simulink model "BCM_C1A_EcuMonitor_4"  (Simulink 9.2)
settings: Solver=FixedStepDiscrete  StartTime=0.0  StopTime=5  FixedStep=0.01  RelTol=1e-3
undefined symbols (not defined in the file or in its folder): PRSK_DURATION_UNAVAILABLE_VALUE_CST, SECOND_TO_HUNDRED_MS_CST, TEN_CST, TYP_BCM_PRESOAK_REQUEST, TYP_HEVC_PRESOAK_ACTI_STATUS, TYP_LIN_LOW_LAYER, TYP_LOW_LAYER, TYP_RES_STATUS, TYP_UNDERHOOD_STATE, TYP_WAKE_UP_TYPE, ZERO_CST
libraries: Renault_Library x36, library_BCM x1
(part 1 of 2)
settings Model: Creator=p061584  LastModifiedBy=40005501
settings ConfigSet: Description=Test1
settings DataIOCC: SaveFormat=StructureWithTime  SignalLoggingSaveFormat=Dataset
settings DebuggingCC: SolverPrmCheckMsg=warning  InheritedTsInSrcMsg=none  ParameterPrecisionLossMsg=none
settings HardwareCC: ProdIntDivRoundTo=Zero  ProdEndianess=LittleEndian  ProdHWDeviceType=Generic->32-bit x86 compatible
settings SFSimCC: SimUseLocalCustomCode=on
settings RTWCC: RTWUseLocalCustomCode=on
settings GRTTargetCC: GeneratePreprocessorConditionals=Use local settings
settings ConfigComp: CovMetricSettings=dwe  CovHtmlReporting=off  CovSaveCumulativeToWorkspaceVar=off  CovSaveSingleToWorkspaceVar=off  CovExternalEMLEnable=on  DVMaxTestCaseSteps=500  DVTestSuiteOptimization=CombinedObjectives (Nonlinear Extended)  DVDetectDeadLogic=on  DVDetectActiveLogic=on  DVDetectOutOfBounds=on

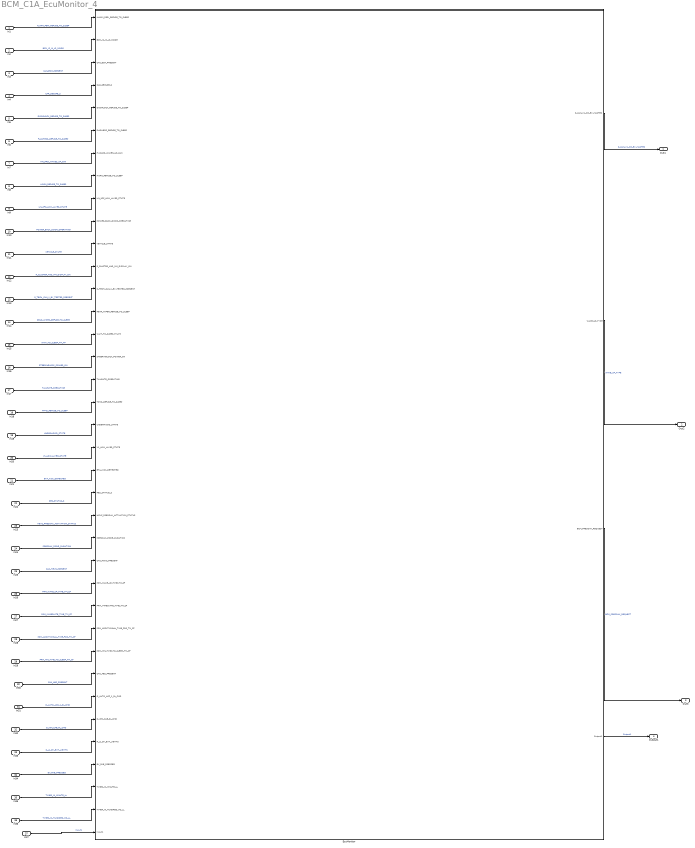
== system BCM_C1A_EcuMonitor_4 ==
  In1 : Inport
  In2 : Inport  Port=2
  In3 : Inport  Port=3
  In4 : Inport  Port=4
  In5 : Inport  Port=5
  In6 : Inport  Port=6
  In7 : Inport  Port=7
  In8 : Inport  Port=8
  In9 : Inport  Port=9
  In10 : Inport  Port=10
  In11 : Inport  Port=11
  In12 : Inport  Port=12
  In13 : Inport  Port=13
  In14 : Inport  Port=14
  In15 : Inport  Port=15
  In16 : Inport  Port=16
  In17 : Inport  Port=17
  In18 : Inport  Port=18
  In19 : Inport  Port=19
  In20 : Inport  Port=20
  In21 : Inport  Port=21
  In22 : Inport  Port=22
  In23 : Inport  Port=23
  In24 : Inport  Port=24
  In25 : Inport  Port=25
  In26 : Inport  Port=26
  In27 : Inport  Port=27
  In28 : Inport  Port=28
  In29 : Inport  Port=29
  In30 : Inport  Port=30
  In31 : Inport  Port=31
  In32 : Inport  Port=32
  In33 : Inport  Port=33
  In34 : Inport  Port=34
  In35 : Inport  Port=35
  In36 : Inport  Port=36
  In37 : Inport  Port=37  OutDataTypeStr=uint8
  EcuMonitor : Subsystem
  Out1 : Outport
  Out2 : Outport  Port=2
  Out3 : Outport  Port=3
  Output1 : Outport  Port=4  OutDataTypeStr=uint8
  wires:
  In30/1 -> EcuMonitor/30(CAN_ABS_PRESENT)  "CAN_ABS_PRESENT"
  In31/1 -> EcuMonitor/31(O_AUTO_ACC_1_RL_CMD)  "O_AUTO_ACC_1_RL_CMD"
  In22/1 -> EcuMonitor/22(RES_STATUS_S)  "RES_STATUS_S"
  In23/1 -> EcuMonitor/23(HEVC_PRESOAK_ACTIVATION_STATUS)  "HEVC_PRESOAK_ACTIVATION_STATUS"
  In24/1 -> EcuMonitor/24(PRESOAK_PROG_DURATION)  "PRESOAK_PROG_DURATION"
  In25/1 -> EcuMonitor/25(CAN_HEVC_PRESENT)  "CAN_HEVC_PRESENT"
  In26/1 -> EcuMonitor/26(PRM_WAKE_UP_TIME_TM_CF)  "PRM_WAKE_UP_TIME_TM_CF"
  In27/1 -> EcuMonitor/27(PRM_IMMEDIATE_TIME_TM_CF)  "PRM_IMMEDIATE_TIME_TM_CF"
  In28/1 -> EcuMonitor/28(PRM_ADDITIONNAL_TIME_FOR_TM_CF)  "PRM_ADDITIONNAL_TIME_FOR_TM_CF"
  In29/1 -> EcuMonitor/29(PRM_MIN_TIME_TO_SLEEP_TM_CF)  "PRM_MIN_TIME_TO_SLEEP_TM_CF"
  In32/1 -> EcuMonitor/32(O_IGN_CAB_RL_CMD)  "O_IGN_CAB_RL_CMD"
  In33/1 -> EcuMonitor/33(R_L1_BY_EXT_LIGHTS)  "R_L1_BY_EXT_LIGHTS"
  In34/1 -> EcuMonitor/34(EV_RKE_PRESSED)  "EV_RKE_PRESSED"
  In35/1 -> EcuMonitor/35(TIMER_IN_MINUTE_LL)  "TIMER_IN_MINUTE_LL"
  In36/1 -> EcuMonitor/36(TIMER_IN_HUNDRED_MS_LL)  "TIMER_IN_HUNDRED_MS_LL"
  In18/1 -> EcuMonitor/18(TPMS_REFUSE_TO_SLEEP)  "TPMS_REFUSE_TO_SLEEP"
  In19/1 -> EcuMonitor/19(UNDERHOOD_STATE)  "UNDERHOOD_STATE"
  In21/1 -> EcuMonitor/21(ETA_KICK_DETECTED)  "ETA_KICK_DETECTED"
  In1/1 -> EcuMonitor/1(ALARM_PERI_REFUSE_TO_SLEEP)  "ALARM_PERI_REFUSE_TO_SLEEP"
  In2/1 -> EcuMonitor/2(BCM_IS_IN_LP_MODE)  "BCM_IS_IN_LP_MODE"
  In3/1 -> EcuMonitor/3(CAN_ECM_PRESENT)  "CAN_ECM_PRESENT"
  In4/1 -> EcuMonitor/4(CAR_SECURE_S)  "CAR_SECURE_S"
  In5/1 -> EcuMonitor/5(DOORLOCK_REFUSE_TO_SLEEP)  "DOORLOCK_REFUSE_TO_SLEEP"
  In6/1 -> EcuMonitor/6(FLASHERS_REFUSE_TO_SLEEP)  "FLASHERS_REFUSE_TO_SLEEP"
  In7/1 -> EcuMonitor/7(HAZARD_WAKES_UP_CAN)  "HAZARD_WAKES_UP_CAN"
  In8/1 -> EcuMonitor/8(HORN_REFUSE_TO_SLEEP)  "HORN_REFUSE_TO_SLEEP"
  In9/1 -> EcuMonitor/9(LIN_NFC_LOW_LAYER_STATE)  "LIN_NFC_LOW_LAYER_STATE"
  In10/1 -> EcuMonitor/10(POWER_BACK_DOOR_OPERATING)  "POWER_BACK_DOOR_OPERATING"
  In11/1 -> EcuMonitor/11(VEHICLE_STATE)  "VEHICLE_STATE"
  In12/1 -> EcuMonitor/12(R_CLUSTER_AND_MM_DISPLAY_ON)  "R_CLUSTER_AND_MM_DISPLAY_ON"
  In13/1 -> EcuMonitor/13(R_TECH_CAN_V_BY_TESTER_PRESENT)  "R_TECH_CAN_V_BY_TESTER_PRESENT"
  In14/1 -> EcuMonitor/14(REAR_WIPER_REFUSE_TO_SLEEP)  "REAR_WIPER_REFUSE_TO_SLEEP"
  In15/1 -> EcuMonitor/15(WAIT_TO_SLEEP_TM_TP)  "WAIT_TO_SLEEP_TM_TP"
  In16/1 -> EcuMonitor/16(STEERINGLOCK_POWER_ON)  "STEERINGLOCK_POWER_ON"
  In17/1 -> EcuMonitor/17(TAILGATE_OPERATING)  "TAILGATE_OPERATING"
  EcuMonitor/1(R_CAN_V1_ON_BY_MASTER) -> Out1/1  "R_CAN_V1_ON_BY_MASTER"
  EcuMonitor/2(WAKE_UP_TYPE) -> Out2/1  "WAKE_UP_TYPE"
  EcuMonitor/3(BCM_PRESOAK_REQUEST) -> Out3/1  "BCM_PRESOAK_REQUEST"
  In20/1 -> EcuMonitor/20(V1_LOW_LAYER_STATE)  "V1_LOW_LAYER_STATE"
  In37/1 -> EcuMonitor/37(Input1)  "Input1"
  EcuMonitor/4(Output1) -> Output1/1  "Output1"

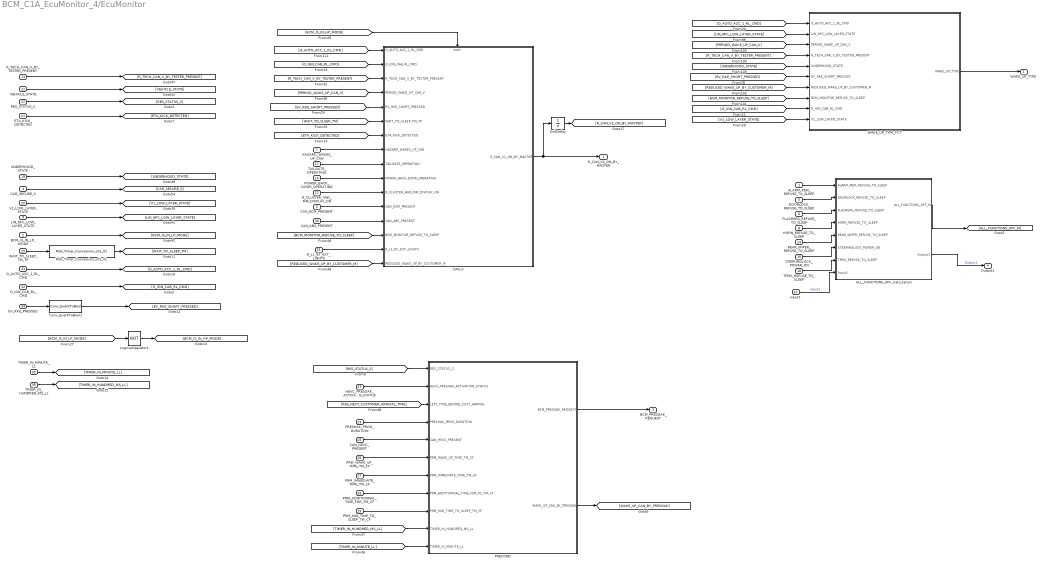
== system BCM_C1A_EcuMonitor_4/EcuMonitor ==
  ALARM_PERI_REFUSE_TO_SLEEP : Inport  OutDataTypeStr=boolean
  BCM_IS_IN_LP_MODE : Inport  Port=2  OutDataTypeStr=boolean
  CAN_ECM_PRESENT : Inport  Port=3  OutDataTypeStr=boolean
  CAR_SECURE_S : Inport  Port=4  OutDataTypeStr=boolean
  DOORLOCK_REFUSE_TO_SLEEP : Inport  Port=5  OutDataTypeStr=boolean
  FLASHERS_REFUSE_TO_SLEEP : Inport  Port=6  OutDataTypeStr=boolean
  HAZARD_WAKES_UP_CAN : Inport  Port=7  OutDataTypeStr=boolean
  HORN_REFUSE_TO_SLEEP : Inport  Port=8  OutDataTypeStr=boolean
  LIN_NFC_LOW_LAYER_STATE : Inport  Port=9  OutDataTypeStr=Enum: TYP_LIN_LOW_LAYER
  POWER_BACK_DOOR_OPERATING : Inport  Port=10  OutDataTypeStr=boolean
  VEHICLE_STATE : Inport  Port=11  OutDataTypeStr=Enum: TYP_VEHICLE_STATE
  R_CLUSTER_AND_MM_DISPLAY_ON : Inport  Port=12  OutDataTypeStr=boolean
  R_TECH_CAN_V_BY_TESTER_PRESENT : Inport  Port=13  OutDataTypeStr=boolean
  REAR_WIPER_REFUSE_TO_SLEEP : Inport  Port=14  OutDataTypeStr=boolean
  WAIT_TO_SLEEP_TM_TP : Inport  Port=15  OutDataTypeStr=uint16
  STEERINGLOCK_POWER_ON : Inport  Port=16  OutDataTypeStr=boolean
  TAILGATE_OPERATING : Inport  Port=17  OutDataTypeStr=boolean
  TPMS_REFUSE_TO_SLEEP : Inport  Port=18  OutDataTypeStr=boolean
  UNDERHOOD_STATE : Inport  Port=19  OutDataTypeStr=Enum: TYP_UNDERHOOD_STATE
  V1_LOW_LAYER_STATE : Inport  Port=20  OutDataTypeStr=Enum: TYP_LOW_LAYER
  ETA_KICK_DETECTED : Inport  Port=21  OutDataTypeStr=boolean
  RES_STATUS_S : Inport  Port=22  OutDataTypeStr=Enum: TYP_RES_STATUS
  HEVC_PRESOAK_ACTIVATION_STATUS : Inport  Port=23  OutDataTypeStr=Enum: TYP_HEVC_PRESOAK_ACTI_STATUS
      settings: AttributesFormatString=Type : %<OutDataTypeStr>
  PRESOAK_PROG_DURATION : Inport  Port=24  OutDataTypeStr=uint8
      settings: AttributesFormatString=Type : %<OutDataTypeStr>
  CAN_HEVC_PRESENT : Inport  Port=25  OutDataTypeStr=boolean
      settings: AttributesFormatString=Type : %<OutDataTypeStr>
  PRM_WAKE_UP_TIME_TM_CF : Inport  Port=26  OutDataTypeStr=uint16
      settings: AttributesFormatString=Type : %<OutDataTypeStr>
  PRM_IMMEDIATE_TIME_TM_CF : Inport  Port=27  OutDataTypeStr=uint16
      settings: AttributesFormatString=Type : %<OutDataTypeStr>
  PRM_ADDITIONNAL_TIME_FOR_TM_CF : Inport  Port=28  OutDataTypeStr=uint16
      settings: AttributesFormatString=Type : %<OutDataTypeStr>
  PRM_MIN_TIME_TO_SLEEP_TM_CF : Inport  Port=29  OutDataTypeStr=uint16
      settings: AttributesFormatString=Type : %<OutDataTypeStr>
  CAN_ABS_PRESENT : Inport  Port=30  OutDataTypeStr=boolean
  O_AUTO_ACC_1_RL_CMD : Inport  Port=31  OutDataTypeStr=boolean
  O_IGN_CAB_RL_CMD : Inport  Port=32  OutDataTypeStr=boolean
  R_L1_BY_EXT_LIGHTS : Inport  Port=33  OutDataTypeStr=boolean
  EV_RKE_PRESSED : Inport  Port=34  OutDataTypeStr=Enum: TYP_EVENT
  TIMER_IN_MINUTE_LL : Inport  Port=35  OutDataTypeStr=uint16
  TIMER_IN_HUNDRED_MS_LL : Inport  Port=36  OutDataTypeStr=uint16
      settings: AttributesFormatString=Type : %<OutDataTypeStr>
  Input1 : Inport  Port=37  OutDataTypeStr=uint8
  ALL_FUNCTIONS_OFF_Calculation : Subsystem
  CAN_V : Subsystem  Description=|
      | RQT_CAN_MANAGEMENT_BCM_420
      | RQT_CAN_MANAGEMENT_BCM_510
      | RQT_CAN_MANAGEMENT_BCM_520
      | RQT_CAN_MANAGEMENT_BCM_700
      | RQT_CAN_MANAGEMENT_BCM_716
      | RQT_EXTLIGHTS_BCM_40
      | RQT_BCM_CSV_4_0
  Conv_EventToBool1 : library_BCM/Modeling/Conv_EventToBool
  LogicalOperator1 : Logic  Operator=NOT  Inputs=7  OutDataTypeStr=boolean
  PRECOND : Subsystem  Description=<binary blob, 195 chars, not shown>
  RSA_Timer_Conversion_v01_01 : Renault_Library/Complex blocks/Timers & Counters/RSA_Timer_Conversion_v01_01  Tag=[LIB]  SAMPLE_TIME_CST=ECUMONITOR_SAMPLE_TIME_CST
      settings: AttributesFormatString=%<MaskType> : Ver : 01.01
  UnitDelay : UnitDelay  SampleTime=-1
      settings: AttributesFormatString=IC = %<X0>
  WAKE_UP_TYPE_FCT : Subsystem  Description=<binary blob, 216 chars, not shown>
  R_CAN_V1_ON_BY_MASTER : Outport  OutDataTypeStr=boolean
      settings: AttributesFormatString=Init :%<InitialOutput>
  WAKE_UP_TYPE : Outport  Port=2  OutDataTypeStr=Enum: TYP_WAKE_UP_TYPE
      settings: AttributesFormatString=Init :%<InitialOutput>
  BCM_PRESOAK_REQUEST : Outport  Port=3  OutDataTypeStr=Enum: TYP_BCM_PRESOAK_REQUEST
      settings: AttributesFormatString=Type : %<OutDataTypeStr>\nInit :%<InitialOutput>
  Output1 : Outport  Port=4  OutDataTypeStr=uint8
      settings: AttributesFormatString=Init :%<InitialOutput>
  wires:
  RES_STATUS_S/1 -> [RES_STATUS_S]
  CAN_ABS_PRESENT/1 -> CAN_V/13(CAN_ABS_PRESENT)
  CAN_ECM_PRESENT/1 -> CAN_V/12(CAN_ECM_PRESENT)
  ETA_KICK_DETECTED/1 -> [ETA_KICK_DETECTED]
  PRECOND/1(BCM_PRESOAK_REQUEST) -> BCM_PRESOAK_REQUEST/1
  PRM_MIN_TIME_TO_SLEEP_TM_CF/1 -> PRECOND/9(PRM_MIN_TIME_TO_SLEEP_TM_CF)
  HEVC_PRESOAK_ACTIVATION_STATUS/1 -> PRECOND/2(HEVC_PRESOAK_ACTIVATION_STATUS)
  [RES_NEXT_CUSTOMER_ARRIVAL_TIME] -> PRECOND/3(LEFT_TIME_BEFORE_CUST_ARRIVAL)
  PRESOAK_PROG_DURATION/1 -> PRECOND/4(PRESOAK_PROG_DURATION)
  CAN_HEVC_PRESENT/1 -> PRECOND/5(CAN_HEVC_PRESENT)
  [RES_STATUS_S] -> PRECOND/1(RES_STATUS_S)
  CAR_SECURE_S/1 -> [CAR_SECURE_S]
  [O_AUTO_ACC_1_RL_CMD] -> CAN_V/1(O_AUTO_ACC_1_RL_CMD)
  VEHICLE_STATE/1 -> [VEHICLE_STATE]
  WAKE_UP_TYPE_FCT/1(WAKE_UP_TYPE) -> WAKE_UP_TYPE/1
  [REDUCED_WAKE_UP_BY_CUSTOMER_M] -> WAKE_UP_TYPE_FCT/7(REDUCED_WAKE_UP_BY_CUSTOMER_M)
  [EV_RKE_SHORT_PRESSED] -> WAKE_UP_TYPE_FCT/6(EV_RKE_SHORT_PRESSED)
  [UNDERHOOD_STATE] -> WAKE_UP_TYPE_FCT/5(UNDERHOOD_STATE)
  [EV_RKE_SHORT_PRESSED] -> CAN_V/5(EV_RKE_SHORT_PRESSED)
  UNDERHOOD_STATE/1 -> [UNDERHOOD_STATE]
  [R_TECH_CAN_V_BY_TESTER_PRESENT] -> WAKE_UP_TYPE_FCT/4(R_TECH_CAN_V_BY_TESTER_PRESENT)
  [PERIOD_WAKE_UP_CAN_V] -> WAKE_UP_TYPE_FCT/3(PERIOD_WAKE_UP_CAN_V)
  [LIN_NFC_LOW_LAYER_STATE] -> WAKE_UP_TYPE_FCT/2(LIN_NFC_LOW_LAYER_STATE)
  [PERIOD_WAKE_UP_CAN_V] -> CAN_V/4(PERIOD_WAKE_UP_CAN_V)
  [R_TECH_CAN_V_BY_TESTER_PRESENT] -> CAN_V/3(R_TECH_CAN_V_BY_TESTER_PRESENT)
  R_TECH_CAN_V_BY_TESTER_PRESENT/1 -> [R_TECH_CAN_V_BY_TESTER_PRESENT]
  WAIT_TO_SLEEP_TM_TP/1 -> RSA_Timer_Conversion_v01_01/1
  R_CLUSTER_AND_MM_DISPLAY_ON/1 -> CAN_V/11(R_CLUSTER_AND_MM_DISPLAY_ON)
  BCM_IS_IN_LP_MODE/1 -> [BCM_IS_IN_LP_MODE]
  LIN_NFC_LOW_LAYER_STATE/1 -> [LIN_NFC_LOW_LAYER_STATE]
  V1_LOW_LAYER_STATE/1 -> [V1_LOW_LAYER_STATE]
  [ETA_KICK_DETECTED] -> CAN_V/7(ETA_KICK_DETECTED)
  CAN_V/1(R_CAN_V1_ON_BY_MASTER) -> UnitDelay/1, R_CAN_V1_ON_BY_MASTER/1
  HAZARD_WAKES_UP_CAN/1 -> CAN_V/8(HAZARD_WAKES_UP_CAN)
  TAILGATE_OPERATING/1 -> CAN_V/9(TAILGATE_OPERATING)
  POWER_BACK_DOOR_OPERATING/1 -> CAN_V/10(POWER_BACK_DOOR_OPERATING)
  PRECOND/2(WAKE_UP_CAN_BY_PRESOAK) -> [WAKE_UP_CAN_BY_PRESOAK]
  [WAIT_TO_SLEEP_TM] -> CAN_V/6(WAIT_TO_SLEEP_TM_TP)
  RSA_Timer_Conversion_v01_01/1 -> [WAIT_TO_SLEEP_TM]
  PRM_WAKE_UP_TIME_TM_CF/1 -> PRECOND/6(PRM_WAKE_UP_TIME_TM_CF)
  PRM_IMMEDIATE_TIME_TM_CF/1 -> PRECOND/7(PRM_IMMEDIATE_TIME_TM_CF)
  PRM_ADDITIONNAL_TIME_FOR_TM_CF/1 -> PRECOND/8(PRM_ADDITIONNAL_TIME_FOR_PC_TM_CF)
  O_AUTO_ACC_1_RL_CMD/1 -> [O_AUTO_ACC_1_RL_CMD]
  [O_AUTO_ACC_1_RL_CMD] -> WAKE_UP_TYPE_FCT/1(O_AUTO_ACC_1_RL_CMD)
  [O_IGN_CAB_RL_CMD] -> WAKE_UP_TYPE_FCT/9(O_IGN_CAB_RL_CMD)
  O_IGN_CAB_RL_CMD/1 -> [O_IGN_CAB_RL_CMD]
  [O_IGN_CAB_RL_CMD] -> CAN_V/2(O_IGN_CAB_RL_CMD)
  [BCM_MONITOR_REFUSE_TO_SLEEP] -> CAN_V/14(BCM_MONITOR_REFUSE_TO_SLEEP)
  R_L1_BY_EXT_LIGHTS/1 -> CAN_V/15(R_L1_BY_EXT_LIGHTS)
  EV_RKE_PRESSED/1 -> Conv_EventToBool1/1
  Conv_EventToBool1/1 -> [EV_RKE_SHORT_PRESSED]
  [BCM_IS_IN_LP_MODE] -> LogicalOperator1/1
  LogicalOperator1/1 -> [BCM_IS_IN_HP_MODE]
  [BCM_IS_IN_HP_MODE] -> CAN_V/Enable
  [REDUCED_WAKE_UP_BY_CUSTOMER_M] -> CAN_V/16(REDUCED_WAKE_UP_BY_CUSTOMER_M)
  [BCM_MONITOR_REFUSE_TO_SLEEP] -> WAKE_UP_TYPE_FCT/8(BCM_MONITOR_REFUSE_TO_SLEEP)
  ALARM_PERI_REFUSE_TO_SLEEP/1 -> ALL_FUNCTIONS_OFF_Calculation/1(ALARM_PERI_REFUSE_TO_SLEEP)
  DOORLOCK_REFUSE_TO_SLEEP/1 -> ALL_FUNCTIONS_OFF_Calculation/2(DOORLOCK_REFUSE_TO_SLEEP)
  FLASHERS_REFUSE_TO_SLEEP/1 -> ALL_FUNCTIONS_OFF_Calculation/3(FLASHERS_REFUSE_TO_SLEEP)
  HORN_REFUSE_TO_SLEEP/1 -> ALL_FUNCTIONS_OFF_Calculation/4(HORN_REFUSE_TO_SLEEP)
  REAR_WIPER_REFUSE_TO_SLEEP/1 -> ALL_FUNCTIONS_OFF_Calculation/5(REAR_WIPER_REFUSE_TO_SLEEP)
  STEERINGLOCK_POWER_ON/1 -> ALL_FUNCTIONS_OFF_Calculation/6(STEERINGLOCK_POWER_ON)
  TPMS_REFUSE_TO_SLEEP/1 -> ALL_FUNCTIONS_OFF_Calculation/7(TPMS_REFUSE_TO_SLEEP)
  ALL_FUNCTIONS_OFF_Calculation/1(ALL_FUNCTIONS_OFF_M) -> [ALL_FUNCTIONS_OFF_M]
  [V1_LOW_LAYER_STATE] -> WAKE_UP_TYPE_FCT/10(V1_LOW_LAYER_STATE)
  TIMER_IN_MINUTE_LL/1 -> [TIMER_IN_MINUTE_LL]
  TIMER_IN_HUNDRED_MS_LL/1 -> [TIMER_IN_HUNDRED_MS_LL]
  [TIMER_IN_HUNDRED_MS_LL] -> PRECOND/10(TIMER_IN_HUNDRED_MS_LL)
  [TIMER_IN_MINUTE_LL] -> PRECOND/11(TIMER_IN_MINUTE_LL)
  UnitDelay/1 -> [R_CAN_V1_ON_BY_MASTER]
  Input1/1 -> ALL_FUNCTIONS_OFF_Calculation/8(Input1)  "Input1"
  ALL_FUNCTIONS_OFF_Calculation/2(Output1) -> Output1/1  "Output1"

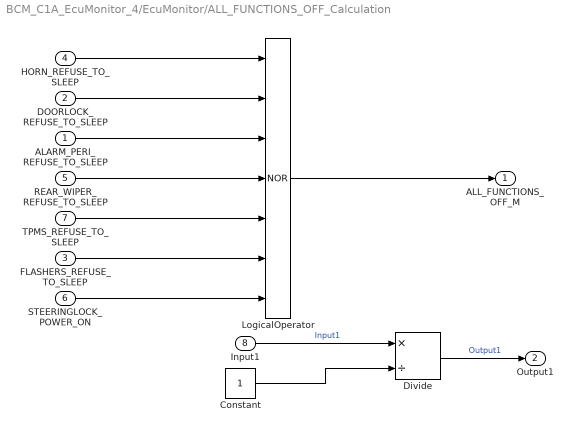
== system BCM_C1A_EcuMonitor_4/EcuMonitor/ALL_FUNCTIONS_OFF_Calculation ==
  ALARM_PERI_REFUSE_TO_SLEEP : Inport  OutDataTypeStr=boolean
  DOORLOCK_REFUSE_TO_SLEEP : Inport  Port=2  OutDataTypeStr=boolean
  FLASHERS_REFUSE_TO_SLEEP : Inport  Port=3  OutDataTypeStr=boolean
  HORN_REFUSE_TO_SLEEP : Inport  Port=4  OutDataTypeStr=boolean
  REAR_WIPER_REFUSE_TO_SLEEP : Inport  Port=5  OutDataTypeStr=boolean
  STEERINGLOCK_POWER_ON : Inport  Port=6  OutDataTypeStr=boolean
  TPMS_REFUSE_TO_SLEEP : Inport  Port=7  OutDataTypeStr=boolean
  Input1 : Inport  Port=8  OutDataTypeStr=uint8
  Constant : Constant
  Divide : Product  Inputs=*/  OutDataTypeStr=uint8
  LogicalOperator : Logic  Operator=NOR  Inputs=7  OutDataTypeStr=boolean
  ALL_FUNCTIONS_OFF_M : Outport
      settings: AttributesFormatString=Init :%<InitialOutput>
  Output1 : Outport  Port=2  OutDataTypeStr=uint8
      settings: AttributesFormatString=Init :%<InitialOutput>
  wires:
  LogicalOperator/1 -> ALL_FUNCTIONS_OFF_M/1
  STEERINGLOCK_POWER_ON/1 -> LogicalOperator/7
  FLASHERS_REFUSE_TO_SLEEP/1 -> LogicalOperator/6
  TPMS_REFUSE_TO_SLEEP/1 -> LogicalOperator/5
  REAR_WIPER_REFUSE_TO_SLEEP/1 -> LogicalOperator/4
  ALARM_PERI_REFUSE_TO_SLEEP/1 -> LogicalOperator/3
  DOORLOCK_REFUSE_TO_SLEEP/1 -> LogicalOperator/2
  HORN_REFUSE_TO_SLEEP/1 -> LogicalOperator/1
  Input1/1 -> Divide/1  "Input1"
  Constant/1 -> Divide/2
  Divide/1 -> Output1/1  "Output1"

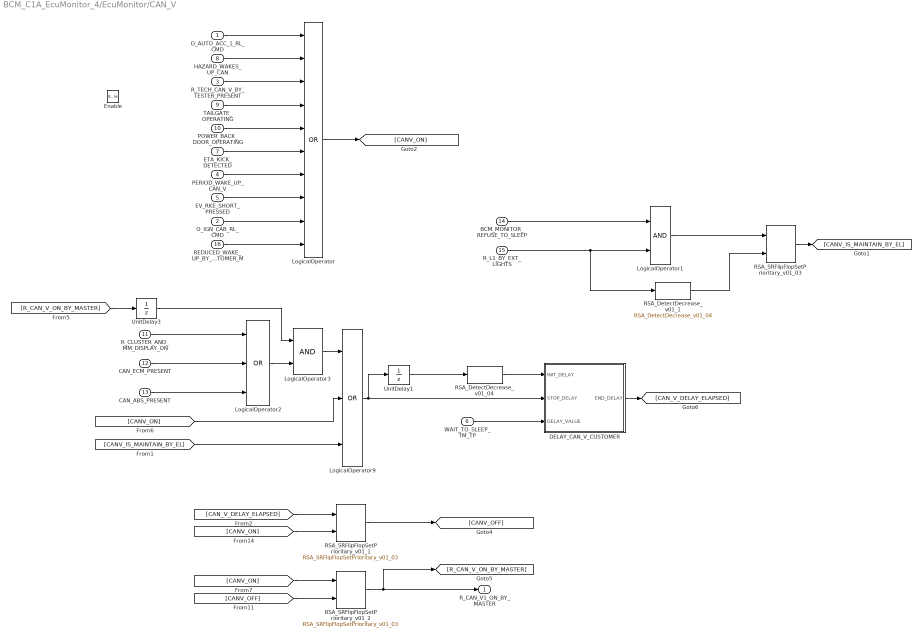
== system BCM_C1A_EcuMonitor_4/EcuMonitor/CAN_V ==
  O_AUTO_ACC_1_RL_CMD : Inport
      settings: AttributesFormatString=Type : %<OutDataTypeStr>
  O_IGN_CAB_RL_CMD : Inport  Port=2
      settings: AttributesFormatString=Type : %<OutDataTypeStr>
  R_TECH_CAN_V_BY_TESTER_PRESENT : Inport  Port=3
      settings: AttributesFormatString=Type : %<OutDataTypeStr>
  PERIOD_WAKE_UP_CAN_V : Inport  Port=4
      settings: AttributesFormatString=Type : %<OutDataTypeStr>
  EV_RKE_SHORT_PRESSED : Inport  Port=5
      settings: AttributesFormatString=Type : %<OutDataTypeStr>
  WAIT_TO_SLEEP_TM_TP : Inport  Port=6
      settings: AttributesFormatString=Type : %<OutDataTypeStr>
  ETA_KICK_DETECTED : Inport  Port=7
      settings: AttributesFormatString=Type : %<OutDataTypeStr>
  HAZARD_WAKES_UP_CAN : Inport  Port=8
      settings: AttributesFormatString=Type : %<OutDataTypeStr>
  TAILGATE_OPERATING : Inport  Port=9
      settings: AttributesFormatString=Type : %<OutDataTypeStr>
  POWER_BACK_DOOR_OPERATING : Inport  Port=10
      settings: AttributesFormatString=Type : %<OutDataTypeStr>
  R_CLUSTER_AND_MM_DISPLAY_ON : Inport  Port=11
      settings: AttributesFormatString=Type : %<OutDataTypeStr>
  CAN_ECM_PRESENT : Inport  Port=12
      settings: AttributesFormatString=Type : %<OutDataTypeStr>
  CAN_ABS_PRESENT : Inport  Port=13
      settings: AttributesFormatString=Type : %<OutDataTypeStr>
  BCM_MONITOR_REFUSE_TO_SLEEP : Inport  Port=14
      settings: AttributesFormatString=Type : %<OutDataTypeStr>
  R_L1_BY_EXT_LIGHTS : Inport  Port=15
      settings: AttributesFormatString=Type : %<OutDataTypeStr>
  REDUCED_WAKE_UP_BY_CUSTOMER_M : Inport  Port=16
      settings: AttributesFormatString=Type : %<OutDataTypeStr>
  Enable : EnablePort
      settings: AttributesFormatString=State : %<StatesWhenEnabling>
  DELAY_CAN_V_CUSTOMER : Subsystem
  LogicalOperator : Logic  Operator=OR  Inputs=10  OutDataTypeStr=boolean
  LogicalOperator1 : Logic  OutDataTypeStr=boolean
  LogicalOperator2 : Logic  Operator=OR  Inputs=3  OutDataTypeStr=boolean
  LogicalOperator3 : Logic  OutDataTypeStr=boolean
  LogicalOperator9 : Logic  Operator=OR  Inputs=3  OutDataTypeStr=boolean
  RSA_DetectDecrease_v01_04 : Renault_Library/Complex blocks/Logic & Bit Operations/RSA_DetectDecrease_v01_04  Tag=[LIB]  chkini=on  vinit=0
      settings: AttributesFormatString=%<MaskType> : Ver : 01.04\nCompare the Input with Initial Value = %<chkini>\nInitial Value : = %<vinit>
  RSA_DetectDecrease_v01_1 : Renault_Library/Complex blocks/Logic & Bit Operations/RSA_DetectDecrease_v01_04  Tag=[LIB]  chkini=on  vinit=0
      settings: AttributesFormatString=%<MaskType> : Ver : 01.04\nCompare the Input with Initial Value = %<chkini>\nInitial Value : = %<vinit>
  RSA_SRFlipFlopSetPrioritary_v01_03 : Renault_Library/Complex blocks/Flip-Flop/RSA_SRFlipFlopSetPrioritary_v01_03  Tag=[LIB]  init=false
      settings: AttributesFormatString=%<MaskType> : Ver : 01.03\n<init=%<init>>
  RSA_SRFlipFlopSetPrioritary_v01_1 : Renault_Library/Complex blocks/Flip-Flop/RSA_SRFlipFlopSetPrioritary_v01_03  Tag=[LIB]  init=false
      settings: AttributesFormatString=%<MaskType> : Ver : 01.03\n<init=%<init>>
  RSA_SRFlipFlopSetPrioritary_v01_2 : Renault_Library/Complex blocks/Flip-Flop/RSA_SRFlipFlopSetPrioritary_v01_03  Tag=[LIB]  init=false
      settings: AttributesFormatString=%<MaskType> : Ver : 01.03\n<init=%<init>>
  UnitDelay1 : UnitDelay  InitialCondition=false  SampleTime=-1
      settings: AttributesFormatString=IC = %<X0>
  UnitDelay3 : UnitDelay  InitialCondition=false  SampleTime=-1
      settings: AttributesFormatString=IC = %<X0>
  R_CAN_V1_ON_BY_MASTER : Outport
      settings: AttributesFormatString=Type : %<OutDataTypeStr>\nInit :%<InitialOutput>
  wires:
  O_AUTO_ACC_1_RL_CMD/1 -> LogicalOperator/1
  [CAN_V_DELAY_ELAPSED] -> RSA_SRFlipFlopSetPrioritary_v01_1/1
  LogicalOperator/1 -> [CANV_ON]
  RSA_SRFlipFlopSetPrioritary_v01_1/1 -> [CANV_OFF]
  [CANV_ON] -> RSA_SRFlipFlopSetPrioritary_v01_1/2
  [CANV_OFF] -> RSA_SRFlipFlopSetPrioritary_v01_2/2
  [CANV_ON] -> RSA_SRFlipFlopSetPrioritary_v01_2/1
  HAZARD_WAKES_UP_CAN/1 -> LogicalOperator/2
  R_TECH_CAN_V_BY_TESTER_PRESENT/1 -> LogicalOperator/3
  TAILGATE_OPERATING/1 -> LogicalOperator/4
  DELAY_CAN_V_CUSTOMER/1(END_DELAY) -> [CAN_V_DELAY_ELAPSED]
  WAIT_TO_SLEEP_TM_TP/1 -> DELAY_CAN_V_CUSTOMER/3(DELAY_VALUE)
  RSA_DetectDecrease_v01_04/1 -> DELAY_CAN_V_CUSTOMER/1(INIT_DELAY)
  [CANV_ON] -> LogicalOperator9/2
  [R_CAN_V_ON_BY_MASTER] -> UnitDelay3/1
  LogicalOperator9/1 -> UnitDelay1/1, DELAY_CAN_V_CUSTOMER/2(STOP_DELAY)
  UnitDelay1/1 -> RSA_DetectDecrease_v01_04/1
  LogicalOperator3/1 -> LogicalOperator9/1
  LogicalOperator2/1 -> LogicalOperator3/2
  CAN_ECM_PRESENT/1 -> LogicalOperator2/2
  CAN_ABS_PRESENT/1 -> LogicalOperator2/3
  R_CLUSTER_AND_MM_DISPLAY_ON/1 -> LogicalOperator2/1
  POWER_BACK_DOOR_OPERATING/1 -> LogicalOperator/5
  ETA_KICK_DETECTED/1 -> LogicalOperator/6
  PERIOD_WAKE_UP_CAN_V/1 -> LogicalOperator/7
  EV_RKE_SHORT_PRESSED/1 -> LogicalOperator/8
  RSA_SRFlipFlopSetPrioritary_v01_2/1 -> [R_CAN_V_ON_BY_MASTER], R_CAN_V1_ON_BY_MASTER/1
  UnitDelay3/1 -> LogicalOperator3/1
  O_IGN_CAB_RL_CMD/1 -> LogicalOperator/9
  R_L1_BY_EXT_LIGHTS/1 -> RSA_DetectDecrease_v01_1/1, LogicalOperator1/2
  BCM_MONITOR_REFUSE_TO_SLEEP/1 -> LogicalOperator1/1
  LogicalOperator1/1 -> RSA_SRFlipFlopSetPrioritary_v01_03/1
  RSA_SRFlipFlopSetPrioritary_v01_03/1 -> [CANV_IS_MAINTAIN_BY_EL]
  RSA_DetectDecrease_v01_1/1 -> RSA_SRFlipFlopSetPrioritary_v01_03/2
  [CANV_IS_MAINTAIN_BY_EL] -> LogicalOperator9/3
  REDUCED_WAKE_UP_BY_CUSTOMER_M/1 -> LogicalOperator/10

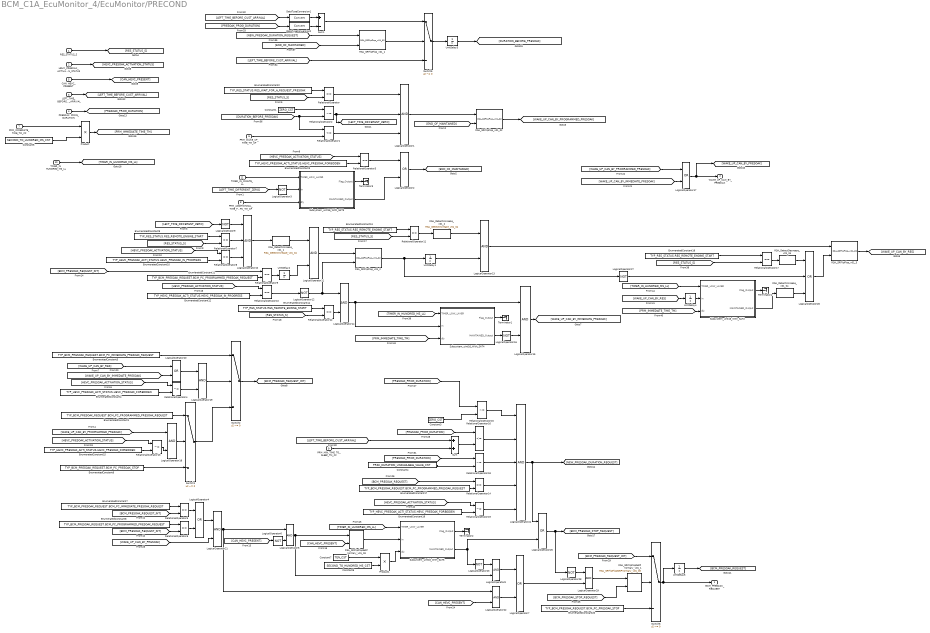
== system BCM_C1A_EcuMonitor_4/EcuMonitor/PRECOND ==
  RES_STATUS_S : Inport
      settings: AttributesFormatString=Type : %<OutDataTypeStr>
  HEVC_PRESOAK_ACTIVATION_STATUS : Inport  Port=2
      settings: AttributesFormatString=Type : %<OutDataTypeStr>
  LEFT_TIME_BEFORE_CUST_ARRIVAL : Inport  Port=3
      settings: AttributesFormatString=Type : %<OutDataTypeStr>
  PRESOAK_PROG_DURATION : Inport  Port=4
      settings: AttributesFormatString=Type : %<OutDataTypeStr>
  CAN_HEVC_PRESENT : Inport  Port=5
      settings: AttributesFormatString=Type : %<OutDataTypeStr>
  PRM_WAKE_UP_TIME_TM_CF : Inport  Port=6
      settings: AttributesFormatString=Type : %<OutDataTypeStr>
  PRM_IMMEDIATE_TIME_TM_CF : Inport  Port=7
      settings: AttributesFormatString=Type : %<OutDataTypeStr>
  PRM_ADDITIONNAL_TIME_FOR_PC_TM_CF : Inport  Port=8
      settings: AttributesFormatString=Type : %<OutDataTypeStr>
  PRM_MIN_TIME_TO_SLEEP_TM_CF : Inport  Port=9
      settings: AttributesFormatString=Type : %<OutDataTypeStr>
  TIMER_IN_HUNDRED_MS_LL : Inport  Port=10
      settings: AttributesFormatString=Type : %<OutDataTypeStr>
  TIMER_IN_MINUTE_LL : Inport  Port=11
      settings: AttributesFormatString=Type : %<OutDataTypeStr>
  Constant1 : Constant  Value=ZERO_CST  OutDataTypeStr=Inherit: Inherit via back propagation
  Constant3 : Constant  Value=ZERO_CST  OutDataTypeStr=uint8  SampleTime=-1
  Constant4 : Constant  Value=PRSK_DURATION_UNAVAILABLE_VALUE_CST  OutDataTypeStr=Inherit: Inherit via back propagation  SampleTime=-1
  Constant5 : Constant  Value=SECOND_TO_HUNDRED_MS_CST  OutDataTypeStr=uint16  SampleTime=-1
  Constant6 : Constant  Value=SECOND_TO_HUNDRED_MS_CST  OutDataTypeStr=uint16  SampleTime=-1
  Constant7 : Constant  Value=TEN_CST  OutDataTypeStr=uint16  SampleTime=-1
  DataTypeConversion1 : DataTypeConversion  RndMeth=Zero
      settings: AttributesFormatString=Saturation:%<SaturateOnIntegerOverflow>
  DataTypeConversion2 : DataTypeConversion  RndMeth=Zero
      settings: AttributesFormatString=Saturation:%<SaturateOnIntegerOverflow>
  EnumeratedConstant{1,8,11,17} (4 alike) : Constant  Value=TYP_BCM_PRESOAK_REQUEST.BCM_PC_PROGRAMMED_PRESOAK_REQUEST  OutDataTypeStr=Enum: TYP_BCM_PRESOAK_REQUEST  SampleTime=-1
  EnumeratedConstant10 : Constant  Value=TYP_HEVC_PRESOAK_ACTI_STATUS.HEVC_PRESOAK_IN_PROGRESS  OutDataTypeStr=Enum: TYP_HEVC_PRESOAK_ACTI_STATUS  SampleTime=-1
  EnumeratedConstant12 : Constant  Value=TYP_HEVC_PRESOAK_ACTI_STATUS.HEVC_PRESOAK_IN_PROGRESS  OutDataTypeStr=Enum: TYP_HEVC_PRESOAK_ACTI_STATUS  SampleTime=-1
  EnumeratedConstant{9,13..14,18} (4 alike) : Constant  Value=TYP_RES_STATUS.RES_REMOTE_ENGINE_START  OutDataTypeStr=Enum: TYP_RES_STATUS  SampleTime=-1
  EnumeratedConstant{3..4,15,19} (4 alike) : Constant  Value=TYP_HEVC_PRESOAK_ACTI_STATUS.HEVC_PRESOAK_FORBIDDEN  OutDataTypeStr=Enum: TYP_HEVC_PRESOAK_ACTI_STATUS  SampleTime=-1
  EnumeratedConstant2 : Constant  Value=TYP_RES_STATUS.RES_WAIT_FOR_A_REQUEST_PRESOAK  OutDataTypeStr=Enum: TYP_RES_STATUS  SampleTime=-1
  EnumeratedConstant20 : Constant  Value=TYP_BCM_PRESOAK_REQUEST.BCM_PC_PRESOAK_STOP  OutDataTypeStr=Enum: TYP_BCM_PRESOAK_REQUEST  SampleTime=-1
  EnumeratedConstant5 : Constant  Value=TYP_BCM_PRESOAK_REQUEST.BCM_PC_IMMEDIATE_PRESOAK_REQUEST  OutDataTypeStr=Enum: TYP_BCM_PRESOAK_REQUEST  SampleTime=-1
  EnumeratedConstant6 : Constant  Value=TYP_BCM_PRESOAK_REQUEST.BCM_PC_PRESOAK_STOP  OutDataTypeStr=Enum: TYP_BCM_PRESOAK_REQUEST  SampleTime=-1
  EnumeratedConstant7 : Constant  Value=TYP_BCM_PRESOAK_REQUEST.BCM_PC_IMMEDIATE_PRESOAK_REQUEST  OutDataTypeStr=Enum: TYP_BCM_PRESOAK_REQUEST  SampleTime=-1
  LogicalOperator1 : Logic  Inputs=3  OutDataTypeStr=boolean
  LogicalOperator10 : Logic  Inputs=3  OutDataTypeStr=boolean
  LogicalOperator{5,8,11,13..15,18..19,21..22,29} (11 alike) : Logic  OutDataTypeStr=boolean
  LogicalOperator{3,6,9,12,16,23,27..28} (8 alike) : Logic  Operator=NOT  OutDataTypeStr=boolean
  LogicalOperator{2,4,7,17,20,25} (6 alike) : Logic  Operator=OR  OutDataTypeStr=boolean
  LogicalOperator24 : Logic  Inputs=5  OutDataTypeStr=boolean
  LogicalOperator26 : Logic  Operator=OR  Inputs=3  OutDataTypeStr=boolean
  Product : Product  OutDataTypeStr=Inherit: Inherit via back propagation  RndMeth=Zero
  Product1 : Product  OutDataTypeStr=Inherit: Inherit via back propagation  RndMeth=Zero
  RSA_DetectDecrease_v01_04 : Renault_Library/Complex blocks/Logic & Bit Operations/RSA_DetectDecrease_v01_04  Tag=[LIB]  chkini=on  vinit=0
      settings: AttributesFormatString=%<MaskType> : Ver : 01.04\nCompare the Input with Initial Value = %<chkini>\nInitial Value : = %<vinit>
  RSA_DetectIncrease_v01_04 : Renault_Library/Complex blocks/Logic & Bit Operations/RSA_DetectIncrease_v01_04  Tag=[LIB]  chkini=on  vinit=0
      settings: AttributesFormatString=%<MaskType> : Ver : 01.04\nCompare the Input with Initial Value = %<chkini>\nInitial Value : = %<vinit>
  RSA_DetectIncrease_v01_1 : Renault_Library/Complex blocks/Logic & Bit Operations/RSA_DetectIncrease_v01_04  Tag=[LIB]  chkini=on  vinit=0
      settings: AttributesFormatString=%<MaskType> : Ver : 01.04\nCompare the Input with Initial Value = %<chkini>\nInitial Value : = %<vinit>
  RSA_DetectIncrease_v01_2 : Renault_Library/Complex blocks/Logic & Bit Operations/RSA_DetectIncrease_v01_04  Tag=[LIB]  chkini=on  vinit=0
      settings: AttributesFormatString=%<MaskType> : Ver : 01.04\nCompare the Input with Initial Value = %<chkini>\nInitial Value : = %<vinit>
  RSA_SRFlipFlopSetPrioritary_v01_03 : Renault_Library/Complex blocks/Flip-Flop/RSA_SRFlipFlopSetPrioritary_v01_03  Tag=[LIB]  init=false
      settings: AttributesFormatString=%<MaskType> : Ver : 01.03\n<init=%<init>>
  RSA_SRFlipFlopSetPrioritary_v01_1 : Renault_Library/Complex blocks/Flip-Flop/RSA_SRFlipFlopSetPrioritary_v01_03  Tag=[LIB]  init=false
      settings: AttributesFormatString=%<MaskType> : Ver : 01.03\n<init=%<init>>
  RSA_SRFlipFlop_v01_02 : Renault_Library/Complex blocks/Flip-Flop/RSA_SRFlipFlop_v01_02  Tag=[LIB]  IC=false
      settings: AttributesFormatString=%<MaskType> : Ver : 01.02\nInitial Condition = %<IC>
  RSA_SRFlipFlop_v01_1 : Renault_Library/Complex blocks/Flip-Flop/RSA_SRFlipFlop_v01_02  Tag=[LIB]  IC=false
      settings: AttributesFormatString=%<MaskType> : Ver : 01.02\nInitial Condition = %<IC>
  RSA_SRFlipFlop_v01_2 : Renault_Library/Complex blocks/Flip-Flop/RSA_SRFlipFlop_v01_02  Tag=[LIB]  IC=false
      settings: AttributesFormatString=%<MaskType> : Ver : 01.02\nInitial Condition = %<IC>
  RSA_SRFlipFlop_v01_3 : Renault_Library/Complex blocks/Flip-Flop/RSA_SRFlipFlop_v01_02  Tag=[LIB]  IC=false
      settings: AttributesFormatString=%<MaskType> : Ver : 01.02\nInitial Condition = %<IC>
  RelationalOperator{,3,5..12,14,17} (12 alike) : RelationalOperator  Operator===  OutDataTypeStr=boolean  RndMeth=Nearest  InputSameDT=on
  RelationalOperator1 : RelationalOperator  Operator=<=  OutDataTypeStr=boolean  RndMeth=Nearest  InputSameDT=on
  RelationalOperator{2,4,13,15,18..19} (6 alike) : RelationalOperator  Operator=~=  OutDataTypeStr=boolean  RndMeth=Nearest  InputSameDT=on
  RelationalOperator16 : RelationalOperator  Operator=<=  OutDataTypeStr=boolean  RndMeth=Nearest  InputSameDT=on
  Subsystem_uint16_With_SAT2 : Subsystem
  Subsystem_uint16_With_SAT3 : Subsystem
  Subsystem_uint16_With_SAT4 : Subsystem
  Subsystem_uint16_With_SAT5 : Subsystem
  Sum : Sum  OutDataTypeStr=Inherit: Inherit via back propagation  RndMeth=Zero  InputSameDT=on
  Sum1 : Sum  Inputs=+-  OutDataTypeStr=Inherit: Inherit via back propagation  RndMeth=Zero  InputSameDT=on
  Switch{1..2,5..6} (4 alike) : Switch  Criteria=u2 ~= 0  RndMeth=Zero  InputSameDT=on
      settings: AttributesFormatString=Criteria=%<Criteria>
  Terminator{1..4} (4 alike) : Terminator
  UnitDelay{1..4} (4 alike) : UnitDelay  InitialCondition=false  SampleTime=-1
      settings: AttributesFormatString=IC = %<X0>
  UnitDelay5 : UnitDelay  InitialCondition=TYP_BCM_PRESOAK_REQUEST.BCM_PC_UNAVAILABLE  SampleTime=-1
      settings: AttributesFormatString=IC = %<X0>
  BCM_PRESOAK_REQUEST : Outport  InitialOutput=TYP_BCM_PRESOAK_REQUEST.BCM_PC_UNAVAILABLE
      settings: AttributesFormatString=Type : %<OutDataTypeStr>\nInit :%<InitialOutput>
  WAKE_UP_CAN_BY_PRESOAK : Outport  Port=2
      settings: AttributesFormatString=Type : %<OutDataTypeStr>\nInit :%<InitialOutput>
  wires:
  PRM_WAKE_UP_TIME_TM_CF/1 -> RelationalOperator1/2
  RSA_SRFlipFlopSetPrioritary_v01_03/1 -> Subsystem_uint16_With_SAT5/2(In)
  [CAN_HEVC_PRESENT] -> RSA_SRFlipFlopSetPrioritary_v01_03/2
  LogicalOperator5/1 -> LogicalOperator8/2, RSA_SRFlipFlopSetPrioritary_v01_03/1
  [CAN_HEVC_PRESENT] -> LogicalOperator6/1
  CAN_HEVC_PRESENT/1 -> [CAN_HEVC_PRESENT]
  LogicalOperator21/1 -> LogicalOperator22/1, LogicalOperator5/1
  LogicalOperator6/1 -> LogicalOperator5/2
  RelationalOperator5/1 -> LogicalOperator4/1
  RelationalOperator6/1 -> LogicalOperator4/2
  [BCM_PRESOAK_REQUEST_INT] -> RelationalOperator6/2
  EnumeratedConstant8/1 -> RelationalOperator6/1
  [BCM_PRESOAK_REQUEST_INT] -> RelationalOperator5/2
  EnumeratedConstant7/1 -> RelationalOperator5/1
  RelationalOperator3/1 -> LogicalOperator2/1
  [HEVC_PRESOAK_ACTIVATION_STATUS] -> RelationalOperator3/1
  HEVC_PRESOAK_ACTIVATION_STATUS/1 -> [HEVC_PRESOAK_ACTIVATION_STATUS]
  Switch2/1 -> [BCM_PRESOAK_REQUEST_INT]
  Switch1/1 -> Switch2/3
  EnumeratedConstant5/1 -> Switch2/1
  [RES_STATUS_S] -> RelationalOperator/2
  RES_STATUS_S/1 -> [RES_STATUS_S]
  [END_OF_MAINTAINED] -> RSA_SRFlipFlop_v01_02/2
  LogicalOperator2/1 -> [END_OF_MAINTAINED]
  EnumeratedConstant3/1 -> RelationalOperator3/2
  RSA_SRFlipFlop_v01_02/1 -> [WAKE_UP_CAN_BY_PROGRAMMED_PRESOAK]
  LogicalOperator1/1 -> RSA_SRFlipFlop_v01_02/1
  LogicalOperator3/1 -> Subsystem_uint16_With_SAT3/2(In)
  [LEFT_TIME_DIFFERENT_ZERO] -> LogicalOperator3/1
  PRM_ADDITIONNAL_TIME_FOR_PC_TM_CF/1 -> Subsystem_uint16_With_SAT3/3(dly)
  EnumeratedConstant1/1 -> Switch1/1
  RelationalOperator/1 -> LogicalOperator1/1
  RelationalOperator1/1 -> LogicalOperator1/3
  RelationalOperator2/1 -> [LEFT_TIME_DIFFERENT_ZERO], LogicalOperator1/2
  Constant1/1 -> RelationalOperator2/1
  EnumeratedConstant2/1 -> RelationalOperator/1
  Subsystem_uint16_With_SAT3/2(MAINTAINED_Output) -> LogicalOperator2/2
  [LEFT_TIME_DIFFERENT_ZERO] -> LogicalOperator9/1
  RelationalOperator7/1 -> LogicalOperator10/2
  [RES_STATUS_S] -> RelationalOperator7/2
  EnumeratedConstant9/1 -> RelationalOperator7/1
  [HEVC_PRESOAK_ACTIVATION_STATUS] -> RelationalOperator8/1
  EnumeratedConstant10/1 -> RelationalOperator8/2
  RelationalOperator8/1 -> LogicalOperator10/3
  LogicalOperator9/1 -> LogicalOperator10/1
  LogicalOperator10/1 -> RSA_DetectIncrease_v01_1/1
  EnumeratedConstant11/1 -> RelationalOperator9/2
  RelationalOperator9/1 -> UnitDelay2/1
  LogicalOperator11/1 -> RSA_SRFlipFlop_v01_2/1
  [HEVC_PRESOAK_ACTIVATION_STATUS] -> RelationalOperator10/1
  EnumeratedConstant12/1 -> RelationalOperator10/2
  RelationalOperator10/1 -> LogicalOperator12/1
  LogicalOperator12/1 -> RSA_SRFlipFlop_v01_2/2, LogicalOperator14/1
  EnumeratedConstant13/1 -> RelationalOperator11/1
  [RES_STATUS_S] -> RelationalOperator11/2
  RelationalOperator12/1 -> LogicalOperator14/2
  EnumeratedConstant14/1 -> RelationalOperator12/1
  [RES_STATUS_S] -> RelationalOperator12/2
  Subsystem_uint16_With_SAT4/2(MAINTAINED_Output) -> LogicalOperator16/1
  LogicalOperator16/1 -> LogicalOperator15/2
  PRM_IMMEDIATE_TIME_TM_CF/1 -> Product/1
  LogicalOperator14/1 -> Subsystem_uint16_With_SAT4/2(In), LogicalOperator15/1
  [HEVC_PRESOAK_ACTIVATION_STATUS] -> RelationalOperator4/1
  EnumeratedConstant4/1 -> RelationalOperator4/2
  EnumeratedConstant6/1 -> Switch1/3
  [HEVC_PRESOAK_ACTIVATION_STATUS] -> RelationalOperator13/1
  EnumeratedConstant15/1 -> RelationalOperator13/2
  RelationalOperator13/1 -> LogicalOperator18/2
  [WAKE_UP_CAN_BY_PROGRAMMED_PRESOAK] -> LogicalOperator18/1
  LogicalOperator18/1 -> Switch1/2
  RelationalOperator4/1 -> LogicalOperator19/2
  LogicalOperator19/1 -> Switch2/2
  LogicalOperator13/1 -> RSA_SRFlipFlop_v01_3/1
  LogicalOperator15/1 -> [WAKE_UP_CAN_BY_IMMEDIATE_PRESOAK]
  [WAKE_UP_CAN_BY_RES] -> LogicalOperator20/1
  [WAKE_UP_CAN_BY_IMMEDIATE_PRESOAK] -> LogicalOperator20/2
  LogicalOperator20/1 -> LogicalOperator19/1
  [WAKE_UP_CAN_BY_IMMEDIATE_PRESOAK] -> LogicalOperator17/2
  [WAKE_UP_CAN_BY_PROGRAMMED_PRESOAK] -> LogicalOperator17/1
  LogicalOperator17/1 -> [WAKE_UP_CAN_BY_PRESOAK], WAKE_UP_CAN_BY_PRESOAK/1
  LogicalOperator4/1 -> LogicalOperator21/1
  [WAKE_UP_CAN_BY_PRESOAK] -> LogicalOperator21/2
  Subsystem_uint16_With_SAT5/1(Flag_Output) -> Terminator2/1
  [CAN_HEVC_PRESENT] -> LogicalOperator22/2
  LogicalOperator22/1 -> LogicalOperator7/2
  Subsystem_uint16_With_SAT5/2(MAINTAINED_Output) -> LogicalOperator25/2, LogicalOperator23/1
  LogicalOperator23/1 -> LogicalOperator8/1
  LogicalOperator8/1 -> LogicalOperator7/1
  EnumeratedConstant17/1 -> RelationalOperator14/2
  [BCM_PRESOAK_REQUEST] -> RelationalOperator14/1
  [PRESOAK_PROG_DURATION] -> RelationalOperator16/1
  LEFT_TIME_BEFORE_CUST_ARRIVAL/1 -> [LEFT_TIME_BEFORE_CUST_ARRIVAL]
  PRESOAK_PROG_DURATION/1 -> [PRESOAK_PROG_DURATION]
  Sum/1 -> RelationalOperator16/2
  [PRESOAK_PROG_DURATION] -> RelationalOperator18/1
  Constant4/1 -> RelationalOperator18/2
  RelationalOperator16/1 -> LogicalOperator24/2
  RelationalOperator18/1 -> LogicalOperator24/3
  RelationalOperator14/1 -> LogicalOperator24/4
  [LEFT_TIME_BEFORE_CUST_ARRIVAL] -> DataTypeConversion1/1
  [PRESOAK_PROG_DURATION] -> DataTypeConversion2/1
  [NEW_PRESOAK_DURATION_REQUEST] -> RSA_SRFlipFlop_v01_1/1
  Sum1/1 -> Switch5/1
  [LEFT_TIME_BEFORE_CUST_ARRIVAL] -> Switch5/3
  Switch5/1 -> UnitDelay3/1
  [DURATION_BEFORE_PRESOAK] -> RelationalOperator1/1, RelationalOperator2/2
  RSA_SRFlipFlop_v01_1/1 -> Switch5/2
  [END_OF_MAINTAINED] -> RSA_SRFlipFlop_v01_1/2
  DataTypeConversion1/1 -> Sum1/1
  DataTypeConversion2/1 -> Sum1/2
  [LEFT_TIME_BEFORE_CUST_ARRIVAL] -> Sum/1
  PRM_MIN_TIME_TO_SLEEP_TM_CF/1 -> Sum/2
  LogicalOperator24/1 -> LogicalOperator25/1, [NEW_PRESOAK_DURATION_REQUEST]
  UnitDelay3/1 -> [DURATION_BEFORE_PRESOAK]
  [BCM_PRESOAK_REQUEST_INT] -> RelationalOperator9/1
  UnitDelay2/1 -> LogicalOperator11/2
  Product/1 -> [PRM_IMMEDIATE_TIME_TM]
  RSA_DetectIncrease_v01_1/1 -> LogicalOperator11/1
  RelationalOperator11/1 -> RSA_DetectIncrease_v01_2/1
  RSA_SRFlipFlop_v01_2/1 -> LogicalOperator27/1, UnitDelay1/1
  UnitDelay1/1 -> LogicalOperator13/2
  RSA_DetectIncrease_v01_2/1 -> LogicalOperator13/1
  RSA_SRFlipFlop_v01_3/1 -> [WAKE_UP_CAN_BY_RES]
  LogicalOperator26/1 -> RSA_SRFlipFlop_v01_3/2
  EnumeratedConstant18/1 -> RelationalOperator17/1
  [RES_STATUS_S] -> RelationalOperator17/2
  RelationalOperator17/1 -> RSA_DetectDecrease_v01_04/1
  RSA_DetectDecrease_v01_04/1 -> LogicalOperator26/1
  LogicalOperator27/1 -> LogicalOperator26/2
  [PRM_IMMEDIATE_TIME_TM] -> Subsystem_uint16_With_SAT2/3(dly)
  Subsystem_uint16_With_SAT2/2(MAINTAINED_Output) -> RSA_DetectIncrease_v01_04/1
  [WAKE_UP_CAN_BY_RES] -> UnitDelay4/1
  RSA_DetectIncrease_v01_04/1 -> LogicalOperator26/3
  UnitDelay4/1 -> Subsystem_uint16_With_SAT2/2(In)
  UnitDelay5/1 -> [BCM_PRESOAK_REQUEST]
  [HEVC_PRESOAK_ACTIVATION_STATUS] -> RelationalOperator19/1
  EnumeratedConstant19/1 -> RelationalOperator19/2
  RelationalOperator19/1 -> LogicalOperator24/5
  LogicalOperator7/1 -> LogicalOperator29/2
  LogicalOperator25/1 -> [BCM_PRESOAK_STOP_REQUEST], LogicalOperator28/1
  [BCM_PRESOAK_REQUEST_INT] -> Switch6/1
  RSA_SRFlipFlopSetPrioritary_v01_1/1 -> Switch6/2
  EnumeratedConstant20/1 -> Switch6/3
  Switch6/1 -> BCM_PRESOAK_REQUEST/1, UnitDelay5/1
  LogicalOperator28/1 -> LogicalOperator29/1
  LogicalOperator29/1 -> RSA_SRFlipFlopSetPrioritary_v01_1/1
  [BCM_PRESOAK_STOP_REQUEST] -> RSA_SRFlipFlopSetPrioritary_v01_1/2
  [PRM_IMMEDIATE_TIME_TM] -> Subsystem_uint16_With_SAT4/3(dly)
  Constant5/1 -> Product/2
  TIMER_IN_HUNDRED_MS_LL/1 -> [TIMER_IN_HUNDRED_MS_LL]
  [TIMER_IN_HUNDRED_MS_LL] -> Subsystem_uint16_With_SAT4/1(TIMER_LOW_LAYER)
  Subsystem_uint16_With_SAT4/1(Flag_Output) -> Terminator1/1
  [TIMER_IN_HUNDRED_MS_LL] -> Subsystem_uint16_With_SAT2/1(TIMER_LOW_LAYER)
  Subsystem_uint16_With_SAT2/1(Flag_Output) -> Terminator4/1
  Constant6/1 -> Product1/2
  Constant7/1 -> Product1/1
  [TIMER_IN_HUNDRED_MS_LL] -> Subsystem_uint16_With_SAT5/1(TIMER_LOW_LAYER)
  Product1/1 -> Subsystem_uint16_With_SAT5/3(dly)
  Subsystem_uint16_With_SAT3/1(Flag_Output) -> Terminator3/1
  TIMER_IN_MINUTE_LL/1 -> Subsystem_uint16_With_SAT3/1(TIMER_LOW_LAYER)
  Constant3/1 -> RelationalOperator15/2
  [PRESOAK_PROG_DURATION] -> RelationalOperator15/1
  RelationalOperator15/1 -> LogicalOperator24/1

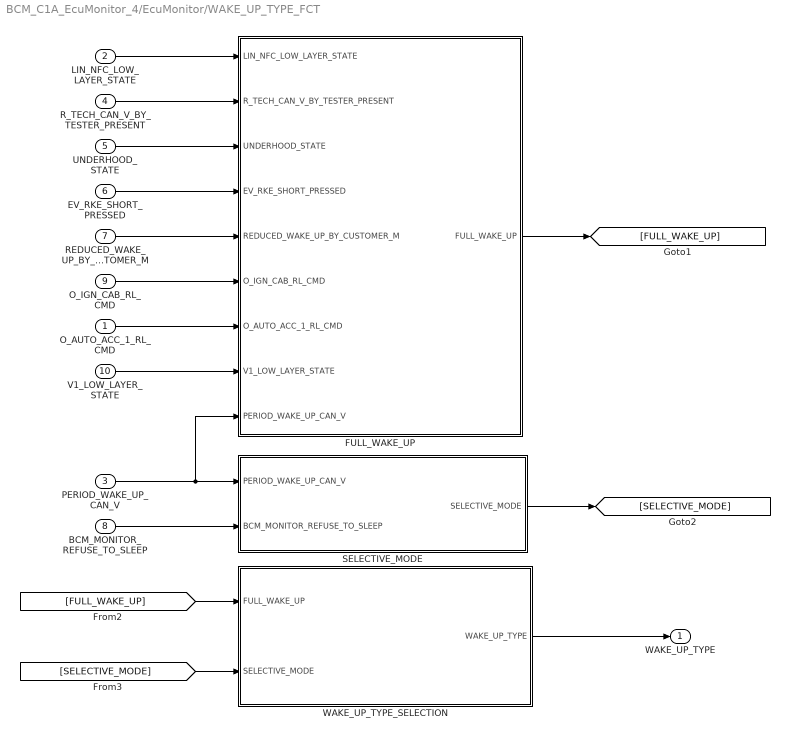
== system BCM_C1A_EcuMonitor_4/EcuMonitor/WAKE_UP_TYPE_FCT ==
  O_AUTO_ACC_1_RL_CMD : Inport
  LIN_NFC_LOW_LAYER_STATE : Inport  Port=2
      settings: AttributesFormatString=Type : %<OutDataTypeStr>
  PERIOD_WAKE_UP_CAN_V : Inport  Port=3
      settings: AttributesFormatString=Type : %<OutDataTypeStr>
  R_TECH_CAN_V_BY_TESTER_PRESENT : Inport  Port=4
      settings: AttributesFormatString=Type : %<OutDataTypeStr>
  UNDERHOOD_STATE : Inport  Port=5
      settings: AttributesFormatString=Type : %<OutDataTypeStr>
  EV_RKE_SHORT_PRESSED : Inport  Port=6
      settings: AttributesFormatString=Type : %<OutDataTypeStr>
  REDUCED_WAKE_UP_BY_CUSTOMER_M : Inport  Port=7
      settings: AttributesFormatString=Type : %<OutDataTypeStr>
  BCM_MONITOR_REFUSE_TO_SLEEP : Inport  Port=8
      settings: AttributesFormatString=Type : %<OutDataTypeStr>
  O_IGN_CAB_RL_CMD : Inport  Port=9
  V1_LOW_LAYER_STATE : Inport  Port=10
      settings: AttributesFormatString=Type : %<OutDataTypeStr>
  FULL_WAKE_UP : Subsystem
  SELECTIVE_MODE : Subsystem
  WAKE_UP_TYPE_SELECTION : Subsystem
  WAKE_UP_TYPE : Outport
      settings: AttributesFormatString=Type : %<OutDataTypeStr>\nInit :%<InitialOutput>
  wires:
  SELECTIVE_MODE/1(SELECTIVE_MODE) -> [SELECTIVE_MODE]
  FULL_WAKE_UP/1(FULL_WAKE_UP) -> [FULL_WAKE_UP]
  PERIOD_WAKE_UP_CAN_V/1 -> FULL_WAKE_UP/9(PERIOD_WAKE_UP_CAN_V), SELECTIVE_MODE/1(PERIOD_WAKE_UP_CAN_V)
  BCM_MONITOR_REFUSE_TO_SLEEP/1 -> SELECTIVE_MODE/2(BCM_MONITOR_REFUSE_TO_SLEEP)
  REDUCED_WAKE_UP_BY_CUSTOMER_M/1 -> FULL_WAKE_UP/5(REDUCED_WAKE_UP_BY_CUSTOMER_M)
  EV_RKE_SHORT_PRESSED/1 -> FULL_WAKE_UP/4(EV_RKE_SHORT_PRESSED)
  UNDERHOOD_STATE/1 -> FULL_WAKE_UP/3(UNDERHOOD_STATE)
  R_TECH_CAN_V_BY_TESTER_PRESENT/1 -> FULL_WAKE_UP/2(R_TECH_CAN_V_BY_TESTER_PRESENT)
  LIN_NFC_LOW_LAYER_STATE/1 -> FULL_WAKE_UP/1(LIN_NFC_LOW_LAYER_STATE)
  WAKE_UP_TYPE_SELECTION/1(WAKE_UP_TYPE) -> WAKE_UP_TYPE/1
  [FULL_WAKE_UP] -> WAKE_UP_TYPE_SELECTION/1(FULL_WAKE_UP)
  [SELECTIVE_MODE] -> WAKE_UP_TYPE_SELECTION/2(SELECTIVE_MODE)
  O_AUTO_ACC_1_RL_CMD/1 -> FULL_WAKE_UP/7(O_AUTO_ACC_1_RL_CMD)
  O_IGN_CAB_RL_CMD/1 -> FULL_WAKE_UP/6(O_IGN_CAB_RL_CMD)
  V1_LOW_LAYER_STATE/1 -> FULL_WAKE_UP/8(V1_LOW_LAYER_STATE)

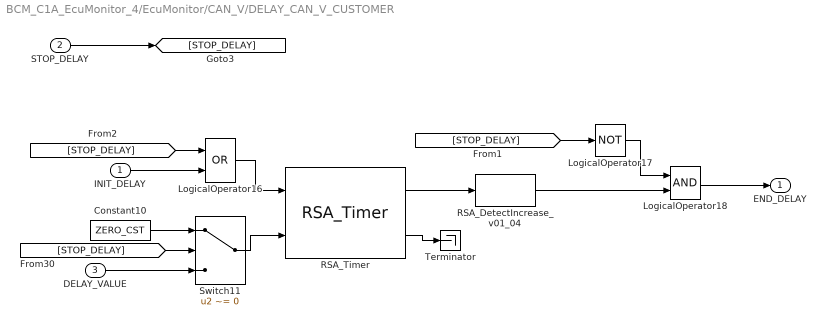
== system BCM_C1A_EcuMonitor_4/EcuMonitor/CAN_V/DELAY_CAN_V_CUSTOMER ==
  INIT_DELAY : Inport
      settings: AttributesFormatString=Type : %<OutDataTypeStr>
  STOP_DELAY : Inport  Port=2
      settings: AttributesFormatString=Type : %<OutDataTypeStr>
  DELAY_VALUE : Inport  Port=3
      settings: AttributesFormatString=Type : %<OutDataTypeStr>
  Constant10 : Constant  Value=ZERO_CST  OutDataTypeStr=Inherit: Inherit via back propagation  SampleTime=-1
  LogicalOperator16 : Logic  Operator=OR  OutDataTypeStr=boolean
  LogicalOperator17 : Logic  Operator=NOT  OutDataTypeStr=boolean
  LogicalOperator18 : Logic  OutDataTypeStr=boolean
  RSA_DetectIncrease_v01_04 : Renault_Library/Complex blocks/Logic & Bit Operations/RSA_DetectIncrease_v01_04  Tag=[LIB]  chkini=on  vinit=0
      settings: AttributesFormatString=%<MaskType> : Ver : 01.04\nCompare the Input with Initial Value = %<chkini>\nInitial Value : = %<vinit>
  RSA_Timer : Renault_Library/Complex blocks/Timers & Counters/RSA_Timer  Tag=[LIB]  timeoutinit=0  initinit=0  st=1
      settings: AttributesFormatString=%<MaskType> : Ver : 01.03\nTimeout output initialisation=%<timeoutinit>\nInit input initialisation=%<initinit>
  Switch11 : Switch  Criteria=u2 ~= 0  RndMeth=Zero  InputSameDT=on
      settings: AttributesFormatString=Criteria=%<Criteria>
  Terminator : Terminator
  END_DELAY : Outport
      settings: AttributesFormatString=Type : %<OutDataTypeStr>\nInit :%<InitialOutput>
  wires:
  RSA_DetectIncrease_v01_04/1 -> LogicalOperator18/2
  LogicalOperator16/1 -> RSA_Timer/1
  INIT_DELAY/1 -> LogicalOperator16/2
  [STOP_DELAY] -> LogicalOperator16/1
  LogicalOperator18/1 -> END_DELAY/1
  LogicalOperator17/1 -> LogicalOperator18/1
  [STOP_DELAY] -> LogicalOperator17/1
  [STOP_DELAY] -> Switch11/2
  STOP_DELAY/1 -> [STOP_DELAY]
  DELAY_VALUE/1 -> Switch11/3
  Switch11/1 -> RSA_Timer/2
  Constant10/1 -> Switch11/1
  RSA_Timer/1 -> RSA_DetectIncrease_v01_04/1
  RSA_Timer/2 -> Terminator/1

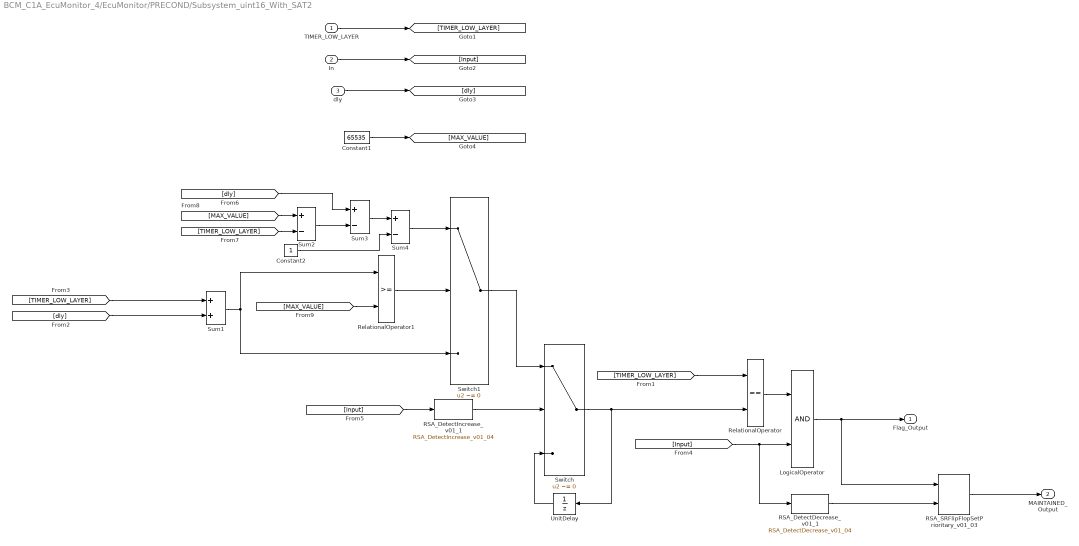
== system BCM_C1A_EcuMonitor_4/EcuMonitor/PRECOND/Subsystem_uint16_With_SAT2 ==
  TIMER_LOW_LAYER : Inport
      settings: AttributesFormatString=Type : %<OutDataTypeStr>
  In : Inport  Port=2
      settings: AttributesFormatString=Type : %<OutDataTypeStr>
  dly : Inport  Port=3
      settings: AttributesFormatString=Type : %<OutDataTypeStr>
  Constant1 : Constant  Value=65535  OutDataTypeStr=uint16  SampleTime=-1
  Constant2 : Constant  OutDataTypeStr=uint16  SampleTime=-1
  LogicalOperator : Logic  OutDataTypeStr=boolean
  RSA_DetectDecrease_v01_1 : Renault_Library/Complex blocks/Logic & Bit Operations/RSA_DetectDecrease_v01_04  Tag=[LIB]  chkini=on  vinit=0
      settings: AttributesFormatString=%<MaskType> : Ver : 01.04\nCompare the Input with Initial Value = %<chkini>\nInitial Value : = %<vinit>
  RSA_DetectIncrease_v01_1 : Renault_Library/Complex blocks/Logic & Bit Operations/RSA_DetectIncrease_v01_04  Tag=[LIB]  chkini=on  vinit=0
      settings: AttributesFormatString=%<MaskType> : Ver : 01.04\nCompare the Input with Initial Value = %<chkini>\nInitial Value : = %<vinit>
  RSA_SRFlipFlopSetPrioritary_v01_03 : Renault_Library/Complex blocks/Flip-Flop/RSA_SRFlipFlopSetPrioritary_v01_03  Tag=[LIB]  init=false
      settings: AttributesFormatString=%<MaskType> : Ver : 01.03\n<init=%<init>>
  RelationalOperator : RelationalOperator  Operator===  OutDataTypeStr=boolean  RndMeth=Nearest  InputSameDT=on
  RelationalOperator1 : RelationalOperator  OutDataTypeStr=boolean  RndMeth=Nearest  InputSameDT=on
  Sum1 : Sum  AccumDataTypeStr=uint16  OutDataTypeStr=Inherit: Inherit via back propagation  RndMeth=Zero  SaturateOnIntegerOverflow=on  InputSameDT=on
  Sum2 : Sum  Inputs=+-  AccumDataTypeStr=uint16  OutDataTypeStr=Inherit: Inherit via back propagation  RndMeth=Zero  SaturateOnIntegerOverflow=on  InputSameDT=on
  Sum3 : Sum  Inputs=+-  AccumDataTypeStr=uint16  OutDataTypeStr=Inherit: Inherit via back propagation  RndMeth=Zero  SaturateOnIntegerOverflow=on  InputSameDT=on
  Sum4 : Sum  Inputs=+-  AccumDataTypeStr=uint16  OutDataTypeStr=Inherit: Inherit via back propagation  RndMeth=Zero  SaturateOnIntegerOverflow=on  InputSameDT=on
  Switch : Switch  Criteria=u2 ~= 0  RndMeth=Zero  InputSameDT=on
      settings: AttributesFormatString=Criteria=%<Criteria>
  Switch1 : Switch  Criteria=u2 ~= 0  RndMeth=Zero  InputSameDT=on
      settings: AttributesFormatString=Criteria=%<Criteria>
  UnitDelay : UnitDelay  SampleTime=-1
      settings: AttributesFormatString=IC = %<X0>
  Flag_Output : Outport
      settings: AttributesFormatString=Type : %<OutDataTypeStr>\nInit :%<InitialOutput>
  MAINTAINED_Output : Outport  Port=2
      settings: AttributesFormatString=Type : %<OutDataTypeStr>\nInit :%<InitialOutput>
  wires:
  Switch1/1 -> Switch/1
  Sum4/1 -> Switch1/1
  Constant2/1 -> Sum4/2
  Sum3/1 -> Sum4/1
  Sum2/1 -> Sum3/2
  [dly] -> Sum3/1
  [TIMER_LOW_LAYER] -> Sum2/2
  [dly] -> Sum1/2
  dly/1 -> [dly]
  RelationalOperator1/1 -> Switch1/2
  Switch/1 -> UnitDelay/1, RelationalOperator/2
  Sum1/1 -> RelationalOperator1/1, Switch1/3
  LogicalOperator/1 -> RSA_SRFlipFlopSetPrioritary_v01_03/1, Flag_Output/1
  RSA_DetectIncrease_v01_1/1 -> Switch/2
  [Input] -> RSA_DetectIncrease_v01_1/1
  In/1 -> [Input]
  TIMER_LOW_LAYER/1 -> [TIMER_LOW_LAYER]
  [TIMER_LOW_LAYER] -> Sum1/1
  UnitDelay/1 -> Switch/3
  [TIMER_LOW_LAYER] -> RelationalOperator/1
  [Input] -> RSA_DetectDecrease_v01_1/1, LogicalOperator/2
  RelationalOperator/1 -> LogicalOperator/1
  RSA_DetectDecrease_v01_1/1 -> RSA_SRFlipFlopSetPrioritary_v01_03/2
  RSA_SRFlipFlopSetPrioritary_v01_03/1 -> MAINTAINED_Output/1
  Constant1/1 -> [MAX_VALUE]
  [MAX_VALUE] -> Sum2/1
  [MAX_VALUE] -> RelationalOperator1/2

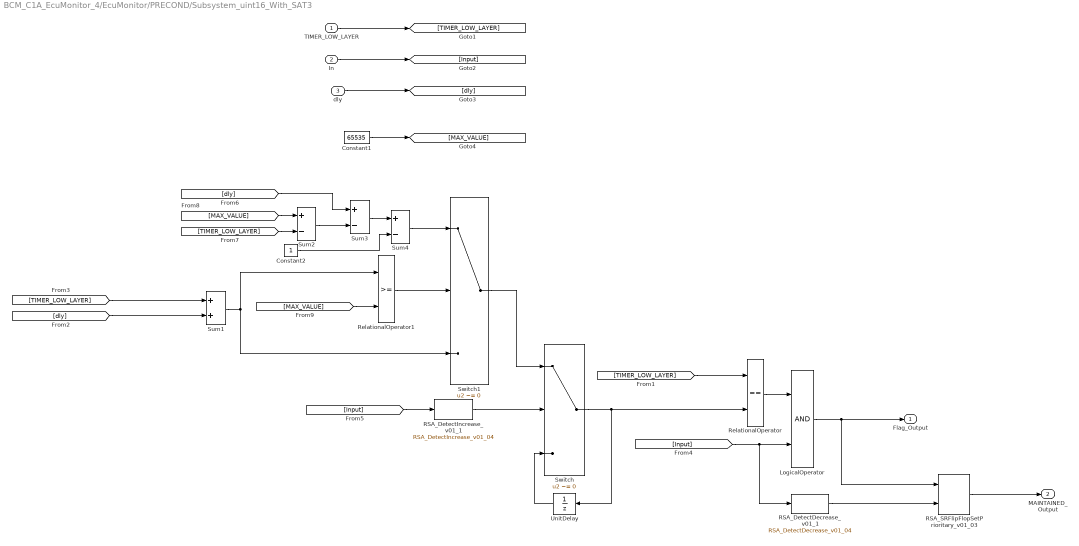
== system BCM_C1A_EcuMonitor_4/EcuMonitor/PRECOND/Subsystem_uint16_With_SAT3 ==
  TIMER_LOW_LAYER : Inport
      settings: AttributesFormatString=Type : %<OutDataTypeStr>
  In : Inport  Port=2
      settings: AttributesFormatString=Type : %<OutDataTypeStr>
  dly : Inport  Port=3
      settings: AttributesFormatString=Type : %<OutDataTypeStr>
  Constant1 : Constant  Value=65535  OutDataTypeStr=uint16  SampleTime=-1
  Constant2 : Constant  OutDataTypeStr=uint16  SampleTime=-1
  LogicalOperator : Logic  OutDataTypeStr=boolean
  RSA_DetectDecrease_v01_1 : Renault_Library/Complex blocks/Logic & Bit Operations/RSA_DetectDecrease_v01_04  Tag=[LIB]  chkini=on  vinit=0
      settings: AttributesFormatString=%<MaskType> : Ver : 01.04\nCompare the Input with Initial Value = %<chkini>\nInitial Value : = %<vinit>
  RSA_DetectIncrease_v01_1 : Renault_Library/Complex blocks/Logic & Bit Operations/RSA_DetectIncrease_v01_04  Tag=[LIB]  chkini=on  vinit=0
      settings: AttributesFormatString=%<MaskType> : Ver : 01.04\nCompare the Input with Initial Value = %<chkini>\nInitial Value : = %<vinit>
  RSA_SRFlipFlopSetPrioritary_v01_03 : Renault_Library/Complex blocks/Flip-Flop/RSA_SRFlipFlopSetPrioritary_v01_03  Tag=[LIB]  init=false
      settings: AttributesFormatString=%<MaskType> : Ver : 01.03\n<init=%<init>>
  RelationalOperator : RelationalOperator  Operator===  OutDataTypeStr=boolean  RndMeth=Nearest  InputSameDT=on
  RelationalOperator1 : RelationalOperator  OutDataTypeStr=boolean  RndMeth=Nearest  InputSameDT=on
  Sum1 : Sum  AccumDataTypeStr=uint16  OutDataTypeStr=Inherit: Inherit via back propagation  RndMeth=Zero  SaturateOnIntegerOverflow=on  InputSameDT=on
  Sum2 : Sum  Inputs=+-  AccumDataTypeStr=uint16  OutDataTypeStr=Inherit: Inherit via back propagation  RndMeth=Zero  SaturateOnIntegerOverflow=on  InputSameDT=on
  Sum3 : Sum  Inputs=+-  AccumDataTypeStr=uint16  OutDataTypeStr=Inherit: Inherit via back propagation  RndMeth=Zero  SaturateOnIntegerOverflow=on  InputSameDT=on
  Sum4 : Sum  Inputs=+-  AccumDataTypeStr=uint16  OutDataTypeStr=Inherit: Inherit via back propagation  RndMeth=Zero  SaturateOnIntegerOverflow=on  InputSameDT=on
  Switch : Switch  Criteria=u2 ~= 0  RndMeth=Zero  InputSameDT=on
      settings: AttributesFormatString=Criteria=%<Criteria>
  Switch1 : Switch  Criteria=u2 ~= 0  RndMeth=Zero  InputSameDT=on
      settings: AttributesFormatString=Criteria=%<Criteria>
  UnitDelay : UnitDelay  SampleTime=-1
      settings: AttributesFormatString=IC = %<X0>
  Flag_Output : Outport
      settings: AttributesFormatString=Type : %<OutDataTypeStr>\nInit :%<InitialOutput>
  MAINTAINED_Output : Outport  Port=2
      settings: AttributesFormatString=Type : %<OutDataTypeStr>\nInit :%<InitialOutput>
  wires:
  Switch1/1 -> Switch/1
  Sum4/1 -> Switch1/1
  Constant2/1 -> Sum4/2
  Sum3/1 -> Sum4/1
  Sum2/1 -> Sum3/2
  [dly] -> Sum3/1
  [TIMER_LOW_LAYER] -> Sum2/2
  [dly] -> Sum1/2
  dly/1 -> [dly]
  RelationalOperator1/1 -> Switch1/2
  Switch/1 -> UnitDelay/1, RelationalOperator/2
  Sum1/1 -> RelationalOperator1/1, Switch1/3
  LogicalOperator/1 -> RSA_SRFlipFlopSetPrioritary_v01_03/1, Flag_Output/1
  RSA_DetectIncrease_v01_1/1 -> Switch/2
  [Input] -> RSA_DetectIncrease_v01_1/1
  In/1 -> [Input]
  TIMER_LOW_LAYER/1 -> [TIMER_LOW_LAYER]
  [TIMER_LOW_LAYER] -> Sum1/1
  UnitDelay/1 -> Switch/3
  [TIMER_LOW_LAYER] -> RelationalOperator/1
  [Input] -> RSA_DetectDecrease_v01_1/1, LogicalOperator/2
  RelationalOperator/1 -> LogicalOperator/1
  RSA_DetectDecrease_v01_1/1 -> RSA_SRFlipFlopSetPrioritary_v01_03/2
  RSA_SRFlipFlopSetPrioritary_v01_03/1 -> MAINTAINED_Output/1
  Constant1/1 -> [MAX_VALUE]
  [MAX_VALUE] -> Sum2/1
  [MAX_VALUE] -> RelationalOperator1/2
